simulink model "ss"  (R2020b)
settings: Solver=VariableStepAuto  StartTime=0.0  StopTime=5  RelTol=1e-3
values from neighbouring files (symbols this model uses):
  A1 = [ ... (first row only)    [script_exp8.m]
  B1 = [0 -m*g*d/L/(J/R^2+m)]'    [script_exp8.m]
  C1 = [1 0]    [script_exp8.m]
  x10 = [0 0]'    [script_exp8.m]
settings Model: Creator=lucas  LastModifiedBy=lucas

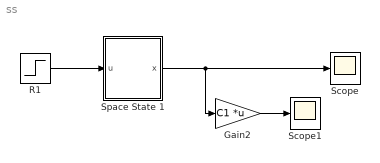
== system ss ==
  Gain2 : Gain  Gain=C1  Multiplication=Matrix(K*u)
  R1 : Step  Time=0  SampleTime=0
  Scope : Scope
  Scope1 : Scope
  Space State 1 : Subsystem
  wires:
  Space State 1/1(x) -> Gain2/1, Scope/1
  R1/1 -> Space State 1/1(u)
  Gain2/1 -> Scope1/1

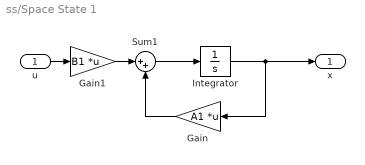
== system ss/Space State 1 ==
  u : Inport
  Gain : Gain  Gain=A1  Multiplication=Matrix(K*u)
  Gain1 : Gain  Gain=B1  Multiplication=Matrix(K*u)
  Integrator : Integrator  InitialCondition=x10
  Sum1 : Sum  Inputs=|++
  x : Outport
  wires:
  Sum1/1 -> Integrator/1
  Gain1/1 -> Sum1/1
  Integrator/1 -> x/1, Gain/1
  u/1 -> Gain1/1
  Gain/1 -> Sum1/2
